simulink model "modello_linearizzazione"  (R2023b)
settings: Solver=VariableStepAuto  StartTime=0.0  StopTime=100  RelTol=1e-3
values from neighbouring files (symbols this model uses):
  alpha_0 = 80 * pi/180    (= 1.3962634016)    [carroponte_controllo.m]
  alpha_dot_0 = 0    [carroponte_controllo.m]
  cc = 5000    [carroponte_controllo.m]
  cm = 100    [carroponte_controllo.m]
  g = 9.81    [carroponte_controllo.m]
  L = 2.5    [carroponte_controllo.m]
  mc = 300    [carroponte_controllo.m]
  mm = 1000    [carroponte_controllo.m]
  xc_0 = 0    [carroponte_controllo.m]
  xc_dot_0 = 0    [carroponte_controllo.m]
undefined symbols (not defined in the file or in its folder): dinamica_alpha_live
libraries: simulink x1
settings Model: Creator=fabio  LastModifiedBy=andrearosini
settings OptimizationCC: BlockReduction=off  DefaultParameterBehavior=Inlined  BufferReuse=off  ReuseModelBlockBuffer=off

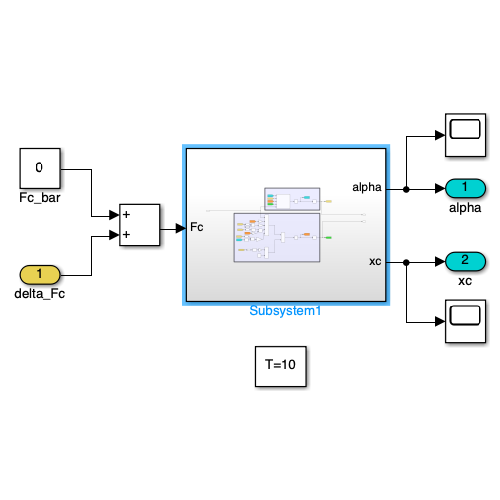
[thumbnail: Simulink's stored preview of the top-level diagram]
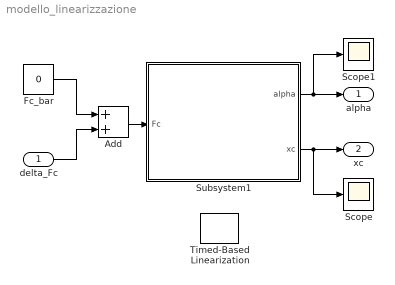
== system modello_linearizzazione ==
  delta_Fc : Inport
  Add : Sum
  Fc_bar : Constant  Value=0
  Scope : Scope
  Scope1 : Scope
  Subsystem1 : Subsystem
  Timed-Based Linearization : simulink/Model-Wide Utilities/Timed-Based Linearization  LinearizationTime=10  SampleTime=0
  alpha : Outport
  xc : Outport  Port=2
  wires:
  Add/1 -> Subsystem1/1(Fc)
  delta_Fc/1 -> Add/2
  Fc_bar/1 -> Add/1
  Subsystem1/1(alpha) -> Scope1/1, alpha/1
  Subsystem1/2(xc) -> Scope/1, xc/1

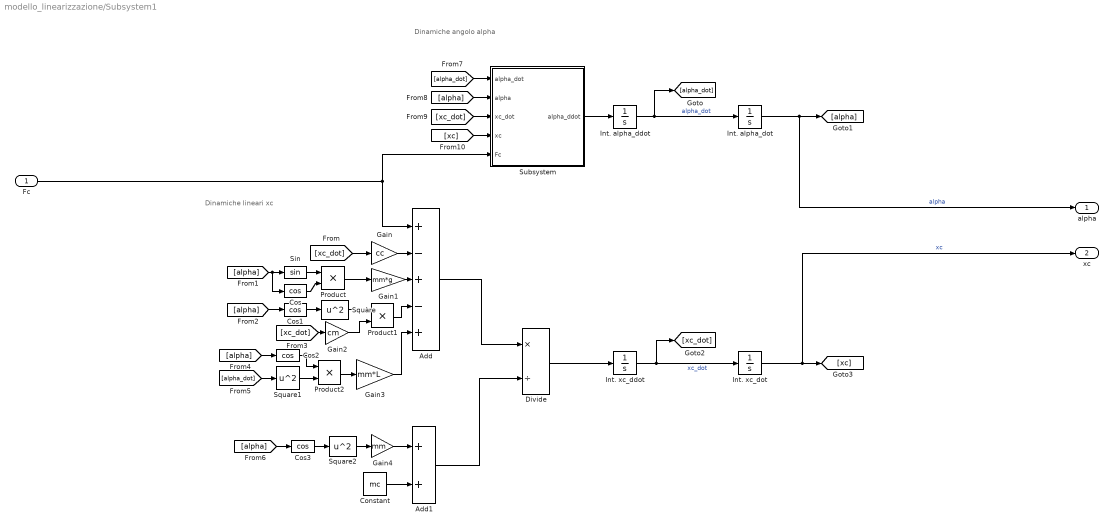
== system modello_linearizzazione/Subsystem1 ==
  note: Dinamiche lineari xc
  note: Dinamiche angolo alpha
  Fc : Inport
  Add : Sum  Inputs=+-+-+
  Add1 : Sum
  Constant : Constant  Value=mc
  Cos{,1..3} (4 alike) : Trigonometry  Operator=cos
  Divide : Product  Inputs=*/
  Gain : Gain  Gain=cc
  Gain1 : Gain  Gain=mm*g
  Gain2 : Gain  Gain=cm
  Gain3 : Gain  Gain=mm*L
  Gain4 : Gain  Gain=mm
  Int. alpha_ddot : Integrator  InitialCondition=alpha_dot_0
  Int. alpha_dot : Integrator  InitialCondition=alpha_0
  Int. xc_ddot : Integrator  InitialCondition=xc_dot_0
  Int. xc_dot : Integrator  InitialCondition=xc_0
  Product : Product
  Product1 : Product
  Product2 : Product
  Sin : Trigonometry
  Square : Math  Operator=square
  Square1 : Math  Operator=square
  Square2 : Math  Operator=square
  Subsystem : Subsystem
  alpha : Outport
  xc : Outport  Port=2
  wires:
  Product/1 -> Gain1/1
  Divide/1 -> Int. xc_ddot/1
  [alpha] -> Cos1/1
  Add/1 -> Divide/1
  Add1/1 -> Divide/2
  [alpha] -> Subsystem/2(alpha)
  Gain1/1 -> Add/3
  Sin/1 -> Product/1
  Cos/1 -> Product/2
  [alpha] -> Cos/1, Sin/1
  Gain3/1 -> Add/5
  Cos1/1 -> Square/1
  Square2/1 -> Gain4/1
  Int. alpha_ddot/1 -> [alpha_dot], Int. alpha_dot/1  "alpha_dot"
  [xc_dot] -> Subsystem/3(xc_dot)
  [alpha_dot] -> Subsystem/1(alpha_dot)
  Int. xc_dot/1 -> xc/1, [xc]  "xc"
  Gain2/1 -> Product1/2
  Constant/1 -> Add1/2
  [xc_dot] -> Gain2/1
  Cos3/1 -> Square2/1
  Square1/1 -> Product2/2
  [alpha_dot] -> Square1/1
  Square/1 -> Product1/1
  Cos2/1 -> Product2/1
  Int. alpha_dot/1 -> alpha/1, [alpha]  "alpha"
  Int. xc_ddot/1 -> [xc_dot], Int. xc_dot/1  "xc_dot"
  [alpha] -> Cos2/1
  [alpha] -> Cos3/1
  Gain/1 -> Add/2
  Product2/1 -> Gain3/1
  Product1/1 -> Add/4
  Subsystem/1(alpha_ddot) -> Int. alpha_ddot/1
  Gain4/1 -> Add1/1
  [xc] -> Subsystem/4(xc)
  [xc_dot] -> Gain/1
  Fc/1 -> Subsystem/5(Fc), Add/1

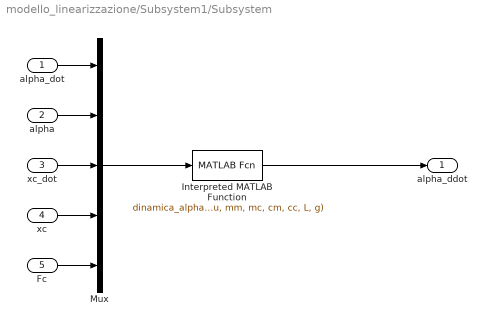
== system modello_linearizzazione/Subsystem1/Subsystem ==
  alpha_dot : Inport
  alpha : Inport  Port=2
  xc_dot : Inport  Port=3
  xc : Inport  Port=4
  Fc : Inport  Port=5
  Interpreted MATLAB Function : MATLABFcn  MATLABFcn=dinamica_alpha_live(u, mm, mc, cm, cc, L, g)
  Mux : Mux  Inputs=5
  alpha_ddot : Outport
  wires:
  alpha_dot/1 -> Mux/1
  alpha/1 -> Mux/2
  xc_dot/1 -> Mux/3
  xc/1 -> Mux/4
  Fc/1 -> Mux/5
  Mux/1 -> Interpreted MATLAB Function/1
  Interpreted MATLAB Function/1 -> alpha_ddot/1
